simulink model "Dead_Zone"  (R2025b)
settings: Solver=FixedStepDiscrete  StartTime=0.0  StopTime=10.0  FixedStep=0.01  RelTol=1e-3
libraries: simulink x2
settings Model: Creator=soura  LastModifiedBy=soura

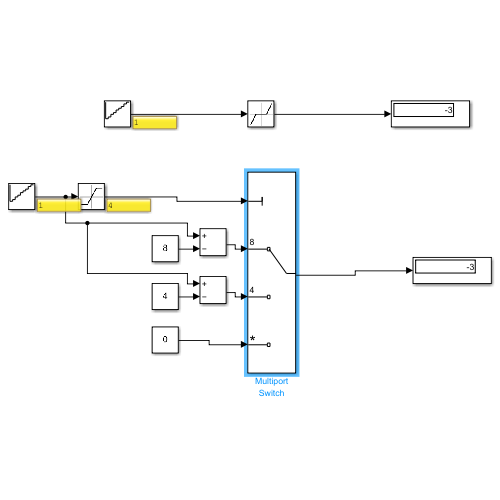
[thumbnail: Simulink's stored preview of the top-level diagram]
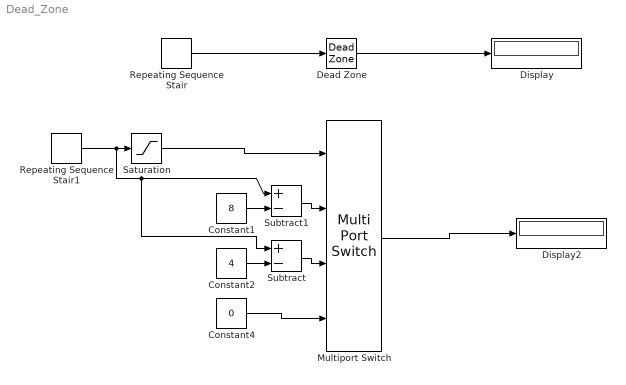
== system Dead_Zone ==
  Constant1 : Constant  Value=8
  Constant2 : Constant  Value=4
  Constant4 : Constant  Value=0
  Dead Zone : DeadZone  LowerValue=4  UpperValue=8  LinearizeAsGain=off
  Display : Display
  Display2 : Display
  Multiport Switch : MultiPortSwitch  DataPortOrder=Specify indices  DataPortIndices={8,4}  DataPortForDefault=Additional data port  DiagnosticForDefault=None  SaturateOnIntegerOverflow=off  InputSameDT=off
  Repeating Sequence Stair : simulink/Sources/Repeating Sequence Stair  OutValues=[1 2 3 4 5 6 7 8 9].'  tsamp=-1  OutMin=[]  OutMax=[]  OutDataTypeStr=double  OutputDataTypeScalingMode=double  OutDataType=fixdt(0,8)  ConRadixGroup=Best Precision: Vector-wise  OutScaling=2^-12
  Repeating Sequence Stair1 : simulink/Sources/Repeating Sequence Stair  OutValues=[1 2 3 4 5 6 7 8 9].'  tsamp=-1  OutMin=[]  OutMax=[]  OutDataTypeStr=double  OutputDataTypeScalingMode=double  OutDataType=fixdt(0,8)  ConRadixGroup=Best Precision: Vector-wise  OutScaling=2^-12
  Saturation : Saturate  UpperLimit=8  LowerLimit=4
  Subtract : Sum  Inputs=+-
  Subtract1 : Sum  Inputs=+-
  wires:
  Repeating Sequence Stair/1 -> Dead Zone/1
  Dead Zone/1 -> Display/1
  Subtract1/1 -> Multiport Switch/2
  Subtract/1 -> Multiport Switch/3
  Saturation/1 -> Multiport Switch/1
  Constant4/1 -> Multiport Switch/4
  Multiport Switch/1 -> Display2/1
  Constant1/1 -> Subtract1/2
  Constant2/1 -> Subtract/2
  Repeating Sequence Stair1/1 -> Subtract/1, Subtract1/1, Saturation/1
